simulink model "tqdtqr_rebuild_V3"  (R2021b)
settings: Solver=VariableStepAuto  StartTime=0.0  StopTime=10.0  RelTol=1e-3
undefined symbols (not defined in the file): ATQD_AfterTqMinGain_X_Deg, ATQD_APSCreepBaseTqD_X_kph, ATQD_APSCreepBaseTqD_Y_Deg, ATQD_APSCreepBaseTqR_X_kph, ATQD_APSCreepBaseTqR_Y_Deg, ATQD_APSCreepIterm_X_kph, ATQD_APSCreepIterm_Y_kph, ATQD_APSCreepPterm_X_kph, ATQD_APSCreepPterm_Y_kph, ATQD_APSDecReq_X_kph, ATQD_APSDecReq_Y_mps2, ATQD_APSDecReqCMD_X_kph, ATQD_APSDecReqTs_X_pct, ATQD_APSDecTimeGain_X_Deg, ATQD_APSDecTimeGain_Y_s, ATQD_APSReqLowSpd_X_Deg, ATQD_AutoHoldReleaseBPS_X_Deg, ATQD_AWDLoadTrqnsGain_X_kg, ATQD_AWDLoadTrqnsGain_Y_pct, ATQD_BOSEnBPSPosn_X_kph, ATQD_BOSMap_X_rpm, ATQD_BOSMap_Y_pct, ATQD_CreepBaseTqD_X_kph, ATQD_CreepBaseTqD_Y_Deg, ATQD_CreepBaseTqR_X_kph, ATQD_CreepBaseTqR_Y_Deg, ATQD_CreepBPSDisPosn_X_Deg, ATQD_CreepBPSDisPosnR_X_Deg, ATQD_CreepBPSEnPosn_X_Deg, ATQD_CreepBPSEnPosnR_X_Deg, ATQD_CreepDeltaTq_X_kph, ATQD_CreepIterm_X_kph, ATQD_CreepIterm_Y_kph, ATQD_CreepItermMaxLimit_X_pct, ATQD_CreepPreloadTime_X_kph, ATQD_CreepPreloadTq_X_kph, ATQD_CreepPreloadTq_Y_s, ATQD_CreepProtTq_X_Deg, ATQD_CreepPterm_X_kph, ATQD_CreepPterm_Y_kph, ATQD_CreepRrTqSpRat_X_rpm, ATQD_CreepRrTqSpRat_Y_Nm, ATQD_CreepTargetSpdD_X_pct, ATQD_CreepTargetSpdR_X_pct, ATQD_CreepUpLimitTq_X_rpm, ATQD_DecIneOPDHoldEnDelay_X_Deg, ATQD_DecIneOPDHoldEnDelay_Y_bar, ATQD_ECOTqMapD_X_rpm, ATQD_ECOTqMapD_Y_pct, ATQD_EMTqMapD_X_rpm, ATQD_EMTqMapD_Y_pct, ATQD_EOPDTqMapDCon_X_rpm, ATQD_EOPDTqMapDCon_Y_Deg, ATQD_EstInitVehWeight_X_c, ATQD_FAfterTqCMDGain_X_rpm, ATQD_FAfterTqCMDGain_Y_pct, ATQD_ForceLowSpd_X_Deg, ATQD_ForcePLimitSpd_X_Deg, ATQD_FrLossMAPLowV_X_rpm, ATQD_FrLossMAPLowV_Y_Nm ... (+949)
libraries: simulink x235, hcu_lib x208, tqr x63, tqd x6
(part 20 of 37)

== system tqdtqr_rebuild_V3/Input_Convert/Main function/Front//Rear ramp parameters determine/Rear First order filter input tau map and determination ==
  note: Drive mode case
  note: Determine Tq by different case
  VTQD_TqTargetShaftSpd_rpm : Inport
  VTQR_EVDriveMode_enum : Inport  Port=2
  VTQD_RollRegenEnable_flg : Inport  Port=3
  VTQD_TqSourceRr_enum : Inport  Port=4
  VTQR_REDUWhlTqReqSmooth_Nm : Inport  Port=5
  VDHP_ActAPSPosn_pct : Inport  Port=6
  VINP_VehSpeed_kph : Inport  Port=7
  VTQD_LimpHomeAct_flg : Inport  Port=8
  VTQD_EVDriveModeValid_flg : Inport  Port=9
  VTQD_RegenMode_enum : Inport  Port=10
  VVMC_ACCPedalOvrd_flg : Inport  Port=11
  VVMC_CCPedalOvrd_flg : Inport  Port=12
  VTQD_PreLoadHold_flg : Inport  Port=13
  VVMC_ActMaxSlideRate_pct : Inport  Port=14
  VTQD_CreepPrLoadEnable_flg : Inport  Port=15
  VTQD_RDCActive_enum : Inport  Port=16
  VTQR_NoABSREDUWhlTqReq_Nm : Inport  Port=17
  VTQR_RampREDUWhlTqReq_Nm : Inport  Port=18
  VTQR_RrFirstOrderInpTq_Nm : Inport  Port=19
  VTQD_PedAccTqEn_flg : Inport  Port=20
  VTQD_PreLoadPreEn_flg : Inport  Port=21
  VVMC_MSAWhlTqActive_flg : Inport  Port=22
  VINP_RrPTCSActive_flg : Inport  Port=23
  VINP_IVISnowModeCmd_flg : Inport  Port=24
  VTQD_IVIRockModeEn_flg : Inport  Port=25
  VINP_VehicleType_enum : Inport  Port=26
  VTQD_CoordWhlTqDemRr_Nm : Inport  Port=27
  VINP_RearAxlTrqReqDrv_Nm : Inport  Port=28
  VVMC_EstSlope_Deg : Inport  Port=29
  AND : Logic  AllPortsSameDT=off  OutDataTypeStr=boolean
  AND1 : Logic  Inputs=3  AllPortsSameDT=off  OutDataTypeStr=boolean
  AND2 : Logic  Inputs=3  AllPortsSameDT=off  OutDataTypeStr=boolean
  AND3 : Logic  AllPortsSameDT=off  OutDataTypeStr=boolean
  AND4 : Logic  AllPortsSameDT=off  OutDataTypeStr=boolean
  Abs : Abs
  Abs4 : Abs
  Add : Sum  Inputs=+-
  Add1 : Sum  Inputs=+-
  Constant1 : Constant  Value=ENUM_TQSOURCE_APS
  Constant10 : Constant  Value=KTQR_PreLoadTs_c
  Constant12 : Constant  Value=KTQR_ARegenLatchEnTq_Nm
  Constant13 : Constant  Value=KTQR_PreLoadPreEnTs_c
  Constant18 : Constant  Value=ENUM_DRIVEMODE_ECO
  Constant19 : Constant  Value=ENUM_DRIVEMODE_NRM
  Constant2 : Constant  Value=KTQR_DriveModeChangeTq_Nm
  Constant20 : Constant  Value=ENUM_DRIVEMODE_SPORT
  Constant3 : Constant  Value=ENUM_TQSOURCE_CC
  Constant32 : Constant  Value=KTQR_TIPOutTsAPS_pct
  Constant33 : Constant  Value=KTQR_TIPOutTsSpd_kph
  Constant34 : Constant  Value=ENUM_TQSOURCE_ADAS
  Constant5 : Constant  Value=ENUM_RDCACTSTA_NOREQUEST
  Constant7 : Constant  Value=ENUM_TQSOURCE_MSA
  Constant8 : Constant  Value=KTQR_DriveModeCMDTqDev_Nm
  Constant9 : Constant  Value=ENUM_VEHICLETYPE_D31L24
  Delay : Delay  DelayLength=1
  Delay1 : Delay  DelayLength=1
  Delay2 : Delay  DelayLength=1
  Detect Change : simulink/Logic and Bit Operations/Detect Change  vinit=0  OutDataTypeStr=boolean
  Equal16 : RelationalOperator  Operator===  OutDataTypeStr=boolean  RndMeth=Simplest
  Equal17 : RelationalOperator  Operator===  OutDataTypeStr=boolean  RndMeth=Simplest
  Equal19 : RelationalOperator  Operator===  OutDataTypeStr=boolean  RndMeth=Simplest
  Equal2 : RelationalOperator  Operator=~=  OutDataTypeStr=boolean  RndMeth=Simplest
  Equal6 : RelationalOperator  Operator=~=  OutDataTypeStr=boolean  RndMeth=Simplest
  GreaterThan2 : RelationalOperator  OutDataTypeStr=boolean  RndMeth=Simplest
  If : If  NumInputs=7  IfExpression=u1~= 0  ElseIfExpressions=u2 ~= 0, u3 ~= 0,u4 ~= 0,u5 ~= 0,u6 ~= 0
  If1 : If  NumInputs=6  IfExpression=u1~= 0  ElseIfExpressions=u2 ~= 0, u3 ~= 0,u4~=0,u5~=0,u6~=0
  Less Than2 : RelationalOperator  Operator=<=  OutDataTypeStr=boolean  RndMeth=Simplest
  Logical Operator : Logic  AllPortsSameDT=off  OutDataTypeStr=boolean
  Logical Operator1 : Logic  Inputs=3  AllPortsSameDT=off  OutDataTypeStr=boolean
  Logical Operator14 : Logic  Operator=OR  Inputs=5  AllPortsSameDT=off  OutDataTypeStr=boolean
  Logical Operator2 : Logic  AllPortsSameDT=off  OutDataTypeStr=boolean
  Logical Operator3 : Logic  Operator=NOT  AllPortsSameDT=off  OutDataTypeStr=boolean
  Logical Operator8 : Logic  Operator=OR  AllPortsSameDT=off  OutDataTypeStr=boolean
  Logical Operator9 : Logic  Operator=NOT  AllPortsSameDT=off  OutDataTypeStr=boolean
  Merge : Merge  Inputs=7
  Merge3 : Merge  Inputs=7
  NOT : Logic  Operator=NOT  AllPortsSameDT=off  OutDataTypeStr=boolean
  NOT1 : Logic  Operator=NOT  AllPortsSameDT=off  OutDataTypeStr=boolean
  OR2 : Logic  Operator=OR  AllPortsSameDT=off  OutDataTypeStr=boolean
  Relational Operator : RelationalOperator  Operator=>  OutDataTypeStr=boolean  RndMeth=Simplest
  Relational Operator1 : RelationalOperator  Operator=~=  OutDataTypeStr=boolean  RndMeth=Simplest
  Relational Operator2 : RelationalOperator  Operator=<=  OutDataTypeStr=boolean  RndMeth=Simplest
  Relational Operator3 : RelationalOperator  Operator===  OutDataTypeStr=boolean  RndMeth=Simplest
  Relational Operator4 : RelationalOperator  Operator===  OutDataTypeStr=boolean  RndMeth=Simplest
  Relational Operator5 : RelationalOperator  Operator=<  OutDataTypeStr=boolean  RndMeth=Simplest
  Relational Operator6 : RelationalOperator  OutDataTypeStr=boolean  RndMeth=Simplest
  Relational Operator7 : RelationalOperator  Operator===  OutDataTypeStr=boolean  RndMeth=Simplest
  SR_Latch1 : hcu_lib/Basic_Blocks/SR_Latch
  Switch4 : Switch  Criteria=u2 > Threshold
  VTQR_CreepREDUTs_c : Subsystem  TreatAsAtomicUnit=on
  VTQR_ECOREDUTs_c : tqr/TQR/Determine Torque Request/TorqueArbitrament/TorqueSmooth/Rear First order filter input tau map and determination/VTQR_ECOREDUTs_c  SystemSampleTime=-1  VariantActivationTime=update diagram  Latency=0  AutoFrameSizeCalculation=off
  VTQR_ESCAPEREDUTs_c : tqr/TQR/Determine Torque Request/TorqueArbitrament/TorqueSmooth/Rear First order filter input tau map and determination/VTQR_ESCAPEREDUTs_c  SystemSampleTime=-1  VariantActivationTime=update diagram  Latency=0  AutoFrameSizeCalculation=off
  VTQR_LHMREDUTs_c : tqr/TQR/Determine Torque Request/TorqueArbitrament/TorqueSmooth/Rear First order filter input tau map and determination/VTQR_LHMREDUTs_c  SystemSampleTime=-1  VariantActivationTime=update diagram  Latency=0  AutoFrameSizeCalculation=off
  VTQR_NORMALREDUTs_c : tqr/TQR/Determine Torque Request/TorqueArbitrament/TorqueSmooth/Rear First order filter input tau map and determination/VTQR_NORMALREDUTs_c  SystemSampleTime=-1  VariantActivationTime=update diagram  Latency=0  AutoFrameSizeCalculation=off
  VTQR_PreLoadPreEnTs_c : Subsystem  TreatAsAtomicUnit=on
  VTQR_PreLoadTs_c : Subsystem  TreatAsAtomicUnit=on
  VTQR_RDCActiveREDUTs_c : Subsystem  TreatAsAtomicUnit=on
  VTQR_REDUTIPOutTs_c : Subsystem  TreatAsAtomicUnit=on
  VTQR_REDUTs_c : Subsystem  TreatAsAtomicUnit=on
  VTQR_SNOWREDUTs_c : tqr/TQR/Determine Torque Request/TorqueArbitrament/TorqueSmooth/Rear First order filter input tau map and determination/VTQR_SNOWREDUTs_c  SystemSampleTime=-1  VariantActivationTime=update diagram  Latency=0  AutoFrameSizeCalculation=off
  VTQR_SPORTREDUTs_c : tqr/TQR/Determine Torque Request/TorqueArbitrament/TorqueSmooth/Rear First order filter input tau map and determination/VTQR_SPORTREDUTs_c  SystemSampleTime=-1  VariantActivationTime=update diagram  Latency=0  AutoFrameSizeCalculation=off
  VTQR_TCSREDUTs_c : tqr/TQR/Determine Torque Request/TorqueArbitrament/TorqueSmooth/Rear First order filter input tau map and determination/VTQR_TCSREDUTs_c  SystemSampleTime=-1  VariantActivationTime=update diagram  Latency=0  AutoFrameSizeCalculation=off
  VTQR_VMCREDUTs_c : Subsystem  TreatAsAtomicUnit=on
  VTQR_RrFirstOrderInpTs_c : Outport
  wires:
  VINP_RearAxlTrqReqDrv_Nm/1 -> [VINP_RearAxlTrqReqDrv_Nm]
  VTQD_CoordWhlTqDemRr_Nm/1 -> [VTQD_CoordWhlTqDemRr_Nm]
  VINP_VehicleType_enum/1 -> [VINP_VehicleType_enum]
  VINP_IVISnowModeCmd_flg/1 -> [VINP_IVISnowModeCmd_flg]
  VTQD_IVIRockModeEn_flg/1 -> [VTQD_IVIRockModeEn_flg]
  VINP_RrPTCSActive_flg/1 -> [VINP_RrPTCSActive_flg]
  [VTQD_PedAccTqEn_flg] -> Logical Operator14/5
  VVMC_MSAWhlTqActive_flg/1 -> [VVMC_MSAWhlTqActive_flg]
  AND3/1 -> Logical Operator14/4
  [VTQD_TqSourceRr_enum] -> Relational Operator7/1
  Relational Operator7/1 -> AND3/1
  Constant7/1 -> Relational Operator7/2
  [VVMC_MSAWhlTqActive_flg] -> AND3/2
  VTQD_PreLoadPreEn_flg/1 -> [VTQD_PreLoadPreEn_flg]
  VVMC_ActMaxSlideRate_pct/1 -> [VVMC_ActMaxSlideRate_pct]
  VTQD_PedAccTqEn_flg/1 -> [VTQD_PedAccTqEn_flg]
  VTQR_RrFirstOrderInpTq_Nm/1 -> [VTQR_RrFirstOrderInpTq_Nm]
  VTQR_RampREDUWhlTqReq_Nm/1 -> [VTQR_RampREDUWhlTqReq_Nm]
  VTQR_NoABSREDUWhlTqReq_Nm/1 -> [VTQR_NoABSREDUWhlTqReq_Nm]
  VTQD_RDCActive_enum/1 -> [VTQD_RDCActive_enum]
  Relational Operator2/1 -> AND/1
  AND/1 -> [VTQR_RrRDCActiveTs_flg]  "VTQR_RrRDCActiveTs_flg"
  Constant5/1 -> Equal2/2
  Equal2/1 -> AND/2
  [VTQD_RDCActive_enum] -> Equal2/1
  [VTQR_RampREDUWhlTqReq_Nm] -> Relational Operator2/1
  Constant12/1 -> Relational Operator2/2
  [VTQD_CreepPrLoadEnable_flg] -> Logical Operator14/3
  VTQD_CreepPrLoadEnable_flg/1 -> [VTQD_CreepPrLoadEnable_flg]
  VTQD_PreLoadHold_flg/1 -> [VTQD_PreLoadHold_flg]
  Constant32/1 -> Less Than2/2
  [VDHP_ActAPSPosn_pct] -> Less Than2/1
  [VTQD_TqSourceRr_enum] -> Relational Operator3/1
  [VVMC_ACCPedalOvrd_flg] -> NOT/1
  [VVMC_CCPedalOvrd_flg] -> NOT1/1
  Relational Operator1/1 -> AND2/3
  Logical Operator14/1 -> AND1/1
  Constant1/1 -> Relational Operator1/2
  GreaterThan2/1 -> AND2/2
  Constant33/1 -> GreaterThan2/2
  NOT/1 -> AND1/2
  NOT1/1 -> AND1/3
  [VTQD_TqSourceRr_enum] -> Relational Operator1/1
  Less Than2/1 -> AND2/1
  [VTQD_TqSourceRr_enum] -> Relational Operator4/1
  Constant34/1 -> Relational Operator4/2
  Relational Operator4/1 -> Logical Operator14/2
  [VINP_VehSpeed_kph] -> GreaterThan2/1
  Relational Operator3/1 -> Logical Operator14/1
  Constant3/1 -> Relational Operator3/2
  VVMC_CCPedalOvrd_flg/1 -> [VVMC_CCPedalOvrd_flg]
  VVMC_ACCPedalOvrd_flg/1 -> [VVMC_ACCPedalOvrd_flg]
  VTQD_RegenMode_enum/1 -> [VTQD_RegenMode_enum]
  VTQD_EVDriveModeValid_flg/1 -> [VTQD_EVDriveModeValid_flg]
  VTQD_RollRegenEnable_flg/1 -> [VTQD_RollRegenEnable_flg]
  VINP_VehSpeed_kph/1 -> [VINP_VehSpeed_kph]
  VDHP_ActAPSPosn_pct/1 -> [VDHP_ActAPSPosn_pct]
  VTQD_LimpHomeAct_flg/1 -> [VTQD_LimpHomeAct_flg]
  VTQR_REDUWhlTqReqSmooth_Nm/1 -> [VTQR_REDUWhlTqReqSmooth_Nm]
  VTQD_TqSourceRr_enum/1 -> [VTQD_TqSourceRr_enum]
  VTQD_TqTargetShaftSpd_rpm/1 -> [VTQD_TqTargetShaftSpd_rpm]
  VTQR_EVDriveMode_enum/1 -> [VTQR_EVDriveMode_enum]
  AND1/1 -> [VTQD_ADASCreepCondition_flg]
  AND2/1 -> [VTQD_APSCondition_flg]
  [VTQR_RrRDCActiveTs_flg] -> If1/1
  If1/1 -> VTQR_RDCActiveREDUTs_c/Action
  [VTQD_RegenMode_enum] -> VTQR_RDCActiveREDUTs_c/1(VTQD_RegenMode_enum)
  [VVMC_ActMaxSlideRate_pct] -> VTQR_RDCActiveREDUTs_c/2(VVMC_ActMaxSlideRate_pct)
  If1/2 -> VTQR_CreepREDUTs_c/Action
  Logical Operator/1 -> If1/2
  [VTQD_ADASCreepCondition_flg] -> Logical Operator/1
  [VTQD_CreepPrLoadEnable_flg] -> Logical Operator/2
  [VTQR_REDUWhlTqReqSmooth_Nm] -> VTQR_CreepREDUTs_c/1(VTQR_REDUWhlTqReqSmooth_Nm)
  [VTQD_TqTargetShaftSpd_rpm] -> VTQR_CreepREDUTs_c/2(VTQD_TqTargetShaftSpd_rpm)
  [VTQD_ADASCreepCondition_flg] -> Logical Operator2/1
  Logical Operator2/1 -> If1/3
  [VTQD_CreepPrLoadEnable_flg] -> Logical Operator3/1
  Logical Operator3/1 -> Logical Operator2/2
  If1/3 -> VTQR_VMCREDUTs_c/Action
  [VTQR_REDUWhlTqReqSmooth_Nm] -> VTQR_VMCREDUTs_c/1(VTQR_REDUWhlTqReqSmooth_Nm)
  [VTQD_TqTargetShaftSpd_rpm] -> VTQR_VMCREDUTs_c/2(VTQD_TqTargetShaftSpd_rpm)
  [VTQD_APSCondition_flg] -> If1/4
  If1/4 -> VTQR_REDUTIPOutTs_c/Action
  [VTQD_PreLoadHold_flg] -> If1/5
  Constant13/1 -> VTQR_PreLoadPreEnTs_c/1(KTQR_PreLoadPreEnTs_c)
  [VTQD_TqTargetShaftSpd_rpm] -> VTQR_REDUTIPOutTs_c/1(VTQD_TqTargetShaftSpd_rpm)
  [VTQD_PreLoadPreEn_flg] -> If1/6
  If1/6 -> VTQR_PreLoadPreEnTs_c/Action
  Constant10/1 -> VTQR_PreLoadTs_c/1(KTQR_PreLoadTs_c)
  If1/5 -> VTQR_PreLoadTs_c/Action
  VTQR_RDCActiveREDUTs_c/1(VTQR_RDCActiveREDUTs_c) -> [VTQR_RDCActiveREDUTs_c]  "VTQR_RDCActiveREDUTs_c"
  VTQR_CreepREDUTs_c/1(VTQR_CreepREDUTs_c) -> [VTQR_CreepREDUTs_c]  "VTQR_CreepREDUTs_c"
  VTQR_VMCREDUTs_c/1(VTQR_VMCREDUTs_c) -> [VTQR_VMCREDUTs_c]  "VTQR_VMCREDUTs_c"
  VTQR_REDUTIPOutTs_c/1(VTQR_REDUTIPOutTs_c) -> [VTQR_REDUTIPOutTs_c]  "VTQR_REDUTIPOutTs_c"
  VTQR_PreLoadTs_c/1(VTQR_PreLoadTs_c) -> [VTQR_PreLoadTs_c]  "VTQR_PreLoadTs_c"
  VTQR_PreLoadPreEnTs_c/1(VTQR_PreLoadPreEnTs_c) -> [VTQR_PreLoadPreEnTs_c]  "VTQR_PreLoadPreEnTs_c"
  [VTQR_REDUTIPOutTs_c] -> Merge/4
  [VTQR_PreLoadTs_c] -> Merge/5
  [VTQR_PreLoadPreEnTs_c] -> Merge/6
  [VTQR_VMCREDUTs_c] -> Merge/3
  [VTQR_CreepREDUTs_c] -> Merge/2
  [VTQR_RDCActiveREDUTs_c] -> Merge/1
  Merge/1 -> VTQR_RrFirstOrderInpTs_c/1  "VTQR_RrFirstOrderInpTs_c"
  VTQR_SNOWREDUTs_c/1 -> [VTQR_SNOWREDUTs_c]  "VTQR_SNOWREDUTs_c"
  Relational Operator/1 -> Logical Operator1/3
  VTQR_NORMALREDUTs_c/1 -> [VTQR_NORMALREDUTs_c]  "VTQR_NORMALREDUTs_c"
  Equal6/1 -> Logical Operator1/2
  [VINP_RearAxlTrqReqDrv_Nm] -> Relational Operator/2
  VTQR_ESCAPEREDUTs_c/1 -> [VTQR_ESCAPEREDUTs_c]  "VTQR_ESCAPEREDUTs_c"
  Logical Operator1/1 -> If/2
  If/5 -> VTQR_NORMALREDUTs_c/Action
  Equal16/1 -> If/6
  [VTQR_REDUWhlTqReqSmooth_Nm] -> VTQR_NORMALREDUTs_c/1
  VTQR_TCSREDUTs_c/1 -> [VTQR_TCSREDUTs_c]  "VTQR_TCSREDUTs_c"
  [VINP_IVISnowModeCmd_flg] -> If/4
  Equal17/1 -> If/5
  Constant18/1 -> Equal16/2
  [VINP_VehicleType_enum] -> Equal6/1
  [VTQD_IVIRockModeEn_flg] -> If/3
  VTQR_LHMREDUTs_c/1 -> [VTQR_LHMREDUTs_c]  "VTQR_LHMREDUTs_c"
  Logical Operator8/1 -> If/1
  VTQR_SPORTREDUTs_c/1 -> [VTQR_SPORTREDUTs_c]  "VTQR_SPORTREDUTs_c"
  If/7 -> VTQR_SPORTREDUTs_c/Action
  [VTQR_REDUWhlTqReqSmooth_Nm] -> VTQR_SNOWREDUTs_c/1
  [VTQR_EVDriveMode_enum] -> Equal17/1
  If/4 -> VTQR_SNOWREDUTs_c/Action
  VTQR_ECOREDUTs_c/1 -> [VTQR_ECOREDUTs_c]  "VTQR_ECOREDUTs_c"
  [VTQD_CoordWhlTqDemRr_Nm] -> Relational Operator/1
  [VTQD_TqTargetShaftSpd_rpm] -> VTQR_SPORTREDUTs_c/2
  [VTQR_REDUWhlTqReqSmooth_Nm] -> VTQR_TCSREDUTs_c/1
  [VTQD_RollRegenEnable_flg] -> VTQR_ECOREDUTs_c/4
  [VTQD_TqTargetShaftSpd_rpm] -> VTQR_TCSREDUTs_c/2
  [VTQD_RegenMode_enum] -> VTQR_NORMALREDUTs_c/3
  [VTQD_TqTargetShaftSpd_rpm] -> VTQR_NORMALREDUTs_c/2
  If/3 -> VTQR_ESCAPEREDUTs_c/Action
  Constant20/1 -> Equal19/2
  [VTQD_TqTargetShaftSpd_rpm] -> VTQR_ESCAPEREDUTs_c/2
  [VTQR_REDUWhlTqReqSmooth_Nm] -> VTQR_ESCAPEREDUTs_c/1
  [VTQR_EVDriveMode_enum] -> Equal16/1
  If/6 -> VTQR_ECOREDUTs_c/Action
  [VINP_RrPTCSActive_flg] -> Logical Operator1/1
  [VTQD_RegenMode_enum] -> VTQR_SPORTREDUTs_c/3
  [VTQR_REDUWhlTqReqSmooth_Nm] -> VTQR_SPORTREDUTs_c/1
  [VTQD_RegenMode_enum] -> VTQR_ECOREDUTs_c/3
  Equal19/1 -> If/7
  Logical Operator9/1 -> Logical Operator8/2
  [VTQD_TqTargetShaftSpd_rpm] -> VTQR_SNOWREDUTs_c/2
  [VTQR_REDUWhlTqReqSmooth_Nm] -> VTQR_ECOREDUTs_c/1
  [VTQR_REDUWhlTqReqSmooth_Nm] -> VTQR_LHMREDUTs_c/1
  If/1 -> VTQR_LHMREDUTs_c/Action
  [VTQR_EVDriveMode_enum] -> Equal19/1
  [VTQD_TqTargetShaftSpd_rpm] -> VTQR_LHMREDUTs_c/2
  Constant9/1 -> Equal6/2
  [VTQD_EVDriveModeValid_flg] -> Logical Operator9/1
  Constant19/1 -> Equal17/2
  If/2 -> VTQR_TCSREDUTs_c/Action
  [VTQD_TqTargetShaftSpd_rpm] -> VTQR_ECOREDUTs_c/2
  [VTQD_LimpHomeAct_flg] -> Logical Operator8/1
  [VTQR_NORMALREDUTs_c] -> Merge3/5
  Merge3/1 -> Switch4/3
  [VTQR_ECOREDUTs_c] -> Merge3/6
  [VTQR_LHMREDUTs_c] -> Merge3/1
  [VTQR_SNOWREDUTs_c] -> Merge3/4
  [VTQR_RrDrModChangeReset_flg] -> SR_Latch1/2
  SR_Latch1/1 -> Switch4/2, [VTQR_RrDrModTsLatch_flg]  "VTQR_RrDrModLatch_flg"
  [VTQR_EVDriveMode_enum] -> Detect Change/1
  Detect Change/1 -> SR_Latch1/1
  [VTQR_SPORTREDUTs_c] -> Merge3/7
  Delay/1 -> Switch4/1
  [VTQR_TCSREDUTs_c] -> Merge3/2
  Switch4/1 -> [VTQR_REDUTs_c], Delay/1  "VTQR_REDUTs_c"
  [VTQR_ESCAPEREDUTs_c] -> Merge3/3
  Relational Operator5/1 -> OR2/1
  Add/1 -> Abs/1
  Delay2/1 -> AND4/2
  Constant8/1 -> Relational Operator6/2
  Add1/1 -> Abs4/1
  [VTQR_RrFirstOrderInpTq_Nm] -> Add1/2
  [VTQR_RrFirstOrderInpTq_Nm] -> Add/2
  [VTQR_NoABSREDUWhlTqReq_Nm] -> Add/1
  [VTQR_RrDrModTsLatch_flg] -> Delay2/1
  Relational Operator6/1 -> AND4/1
  OR2/1 -> [VTQR_RrDrModChangeReset_flg]
  Constant2/1 -> Relational Operator5/2
  Abs/1 -> Relational Operator5/1
  [VTQR_RrFirstOrderInpTq_Nm] -> Delay1/1
  AND4/1 -> OR2/2
  Abs4/1 -> Relational Operator6/1
  Delay1/1 -> Add1/1
  If1/7 -> VTQR_REDUTs_c/Action
  [VTQR_REDUTs_c] -> VTQR_REDUTs_c/1(VTQR_REDUTs_c)
  VTQR_REDUTs_c/1(VTQR_OutREDUTs_c) -> [VTQR_OutREDUTs_c]  "VTQR_OutREDUTs_c"
  [VTQR_OutREDUTs_c] -> Merge/7
  VVMC_EstSlope_Deg/1 -> [VVMC_EstSlope_Deg]
  [VVMC_EstSlope_Deg] -> VTQR_CreepREDUTs_c/3(VVMC_EstSlope_Deg)

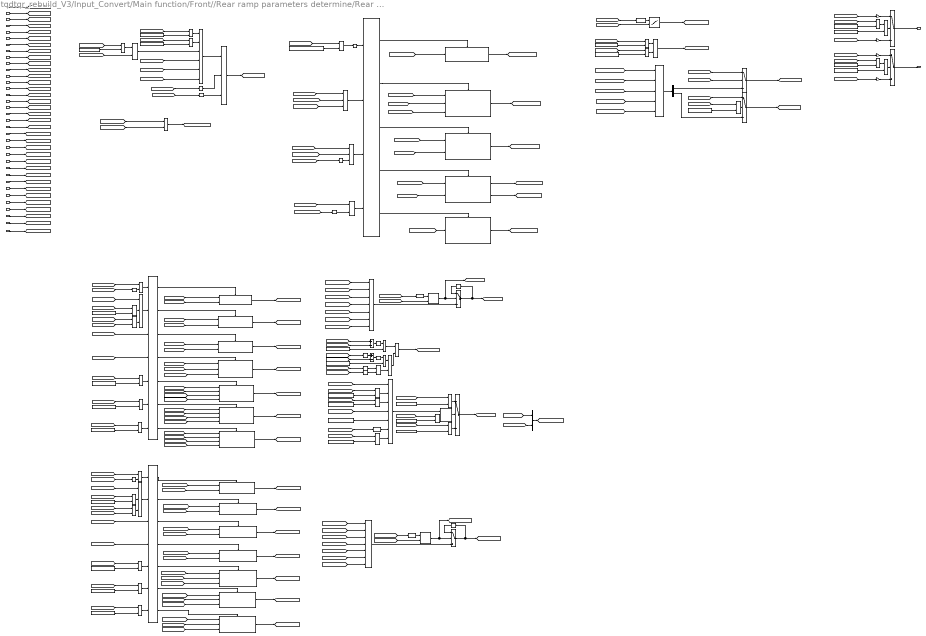
== system tqdtqr_rebuild_V3/Input_Convert/Main function/Front//Rear ramp parameters determine/Rear wheel rate limit determination1 ==
  note: Drive mode case
  note: Determin torque by different cases
  note: Check direction
  note: Merge result and decide final Tq
  VTQR_RrTqZeroTrans_enum : Inport
  VTQD_TqSourceRr_enum : Inport  Port=2
  VTQD_TqTargetShaftSpd_rpm : Inport  Port=3
  VTQD_LimpHomeAct_flg : Inport  Port=4
  VTQR_EVDriveMode_enum : Inport  Port=5
  VDHP_ActAPSPosn_pct : Inport  Port=6
  VTQR_REDUWhlTqReqSmoothDelay_Nm : Inport  Port=7
  VTQD_EVDriveModeValid_flg : Inport  Port=8
  VTQD_RegenMode_enum : Inport  Port=9
  VVMC_ACCPedalOvrd_flg : Inport  Port=10
  VVMC_CCPedalOvrd_flg : Inport  Port=11
  VTQD_CreepPrLoadEnable_flg : Inport  Port=12
  VTQD_RegenTqLimitEn_flg : Inport  Port=13
  VTQD_RDCActive_enum : Inport  Port=14
  VTQD_PreLoadPreEn_flg : Inport  Port=15
  VTQR_NoABSREDUWhlTqReq_Nm : Inport  Port=16
  VTQR_RampREDUWhlTqReq_Nm : Inport  Port=17
  VTQR_RrFirstOrderInpTq_Nm : Inport  Port=18
  VVMC_ActMaxSlideRate_pct : Inport  Port=19
  VTQD_PedAccTqEn_flg : Inport  Port=20
  VVMC_MSAWhlTqActive_flg : Inport  Port=21
  VINP_RrPTCSActive_flg : Inport  Port=22
  VTQD_GearActualPosn_enum : Inport  Port=23
  VINP_IVISnowModeCmd_flg : Inport  Port=24
  VTQD_IVIRockModeEn_flg : Inport  Port=25
  VTQD_RrShaftSpd_rpm : Inport  Port=26
  VVMC_EstSlope_Deg : Inport  Port=27
  VTQD_VehActSpd_kph : Inport  Port=28
  VINP_ACCVehHoldReq_flg : Inport  Port=29
  VPMM_DriveTrainSelect_enum : Inport  Port=30
  VVMC_ADASActive_flg : Inport  Port=31
  VINP_VehicleType_enum : Inport  Port=32
  VTQD_CoordWhlTqDemRr_Nm : Inport  Port=33
  VINP_RearAxlTrqReqDrv_Nm : Inport  Port=34
  VTQD_RrZeroPointIncDec_Nm : Inport  Port=35
  " Relational Operator1" : RelationalOperator  Operator=>  OutDataTypeStr=boolean  RndMeth=Simplest
  " Relational Operator8" : RelationalOperator  Operator=>  OutDataTypeStr=boolean  RndMeth=Simplest
  AND{,2,4..6,9} (6 alike) : Logic  AllPortsSameDT=off  OutDataTypeStr=boolean
  AND7 : Logic  Inputs=7  AllPortsSameDT=off  OutDataTypeStr=boolean
  AND8 : Logic  Inputs=3  AllPortsSameDT=off  OutDataTypeStr=boolean
  Abs : Abs
  Abs4 : Abs
  Add : Sum  Inputs=+-
  Add1 : Sum  Inputs=+-
  Constant : Constant  Value=KTQR_ACCHoldPdovrdGrade_Deg
  Constant11 : Constant  Value=KTQR_ACCHoldPdovrdVeh_kph
  Constant12 : Constant  Value=KTQR_ARegenLatchEnTq_Nm
  Constant13 : Constant  Value=KTQR_ACCHoldPdovrdSW_flg
  Constant14 : Constant  Value=ENUM_DRIVETRAIN_RWD
  Constant15 : Constant  Value=KTQR_ACCHoldPdovrdInc_Nm
  Constant16 : Constant  Value=KTQR_ACCHoldPdovrdInc_Nm
  Constant17 : Constant  Value=ZERO_FLOAT
  Constant18 : Constant  Value=ENUM_GEARACTUALPOSN_R
  Constant19 : Constant  Value=KTQR_NewRampArchSW_flg
  Constant2 : Constant  Value=KTQR_DriveModeChangeTq_Nm
  Constant20 : Constant  Value=ENUM_GEARACTUALPOSN_R
  Constant21 : Constant  Value=KTQR_NewRampArchSW_flg
  Constant22 : Constant  Value=ENUM_DRIVEMODE_ECO
  Constant23 : Constant  Value=ENUM_DRIVEMODE_NRM
  Constant24 : Constant  Value=ENUM_DRIVEMODE_SPORT
  Constant25 : Constant  Value=ENUM_VEHICLETYPE_D31L24
  Constant26 : Constant  Value=ENUM_DRIVEMODE_ECO
  Constant27 : Constant  Value=ENUM_DRIVEMODE_NRM
  Constant28 : Constant  Value=ENUM_DRIVEMODE_SPORT
  Constant29 : Constant  Value=ENUM_VEHICLETYPE_D31L24
  Constant30 : Constant  Value=ENUM_TQSOURCE_ADAS
  Constant4 : Constant  Value=ENUM_TQZEROTRANS_NOZEROTRANS
  Constant5 : Constant  Value=ENUM_RDCACTSTA_NOREQUEST
  Constant6 : Constant  Value=KTQR_RegenTqLimitDecSW_flg
  Constant7 : Constant  Value=ENUM_TQSOURCE_MSA
  Constant8 : Constant  Value=KTQR_DriveModeCMDTqDev_Nm
  Constant9 : Constant  Value=ENUM_TQSOURCE_CC
  Data Type Conversion : DataTypeConversion  OutDataTypeStr=single
  Delay{,1..4} (5 alike) : Delay  DelayLength=1
  Demux : Demux  Outputs=2
  Detect Change : simulink/Logic and Bit Operations/Detect Change  vinit=0  OutDataTypeStr=boolean
  Detect Change1 : simulink/Logic and Bit Operations/Detect Change  vinit=0  OutDataTypeStr=boolean
  Detect Increase : simulink/Logic and Bit Operations/Detect Increase  vinit=0.0  OutDataTypeStr=boolean
  Drive mode : Subsystem  TreatAsAtomicUnit=on
  Equal{,1,5,20..21,23..25,27} (9 alike) : RelationalOperator  Operator===  OutDataTypeStr=boolean  RndMeth=Simplest
  Equal2 : RelationalOperator  Operator=~=  OutDataTypeStr=boolean  RndMeth=Simplest
  Equal3 : RelationalOperator  OutDataTypeStr=boolean  RndMeth=Simplest
  Equal4 : RelationalOperator  Operator=<=  OutDataTypeStr=boolean  RndMeth=Simplest
  Equal6 : RelationalOperator  OutDataTypeStr=boolean  RndMeth=Simplest
  Equal7 : RelationalOperator  Operator=~=  OutDataTypeStr=boolean  RndMeth=Simplest
  Equal8 : RelationalOperator  Operator=~=  OutDataTypeStr=boolean  RndMeth=Simplest
  Gain2 : Gain
  Gain3 : Gain  Gain=-1
  Gain4 : Gain
  Gain5 : Gain  Gain=-1
  If3 : If  NumInputs=4  IfExpression=u1~= 0  ElseIfExpressions=u2 ~= 0, u3 ~= 0, u4~=0
  If4 : If  NumInputs=7  IfExpression=u1~= 0  ElseIfExpressions=u2 ~= 0, u3 ~= 0 ,u4 ~= 0, u5~=0, u6~=0, u7~=0  ShowElse=off
  If5 : If  NumInputs=7  IfExpression=u1~= 0  ElseIfExpressions=u2 ~= 0, u3 ~= 0,u4 ~= 0,u5 ~= 0,u6 ~= 0,u7 ~= 0  ShowElse=off
  Logical Operator{,1..2,5} (4 alike) : Logic  Inputs=3  AllPortsSameDT=off  OutDataTypeStr=boolean
  Logical Operator10 : Logic  Operator=OR  AllPortsSameDT=off  OutDataTypeStr=boolean
  Logical Operator{3,6,9,11,13} (5 alike) : Logic  Operator=NOT  AllPortsSameDT=off  OutDataTypeStr=boolean
  Logical Operator12 : Logic  Operator=OR  AllPortsSameDT=off  OutDataTypeStr=boolean
  Logical Operator4 : Logic  Operator=OR  Inputs=6  AllPortsSameDT=off  OutDataTypeStr=boolean
  Logical Operator8 : Logic  AllPortsSameDT=off  OutDataTypeStr=boolean
  MTQR_AltRDCActiveREDUInc_Z_Nm : Lookup_n-D  BreakpointsForDimension1=ATQR_AltRDCActiveREDUInc_Y_enum  BreakpointsForDimension2=ATQR_AltRDCActiveREDUInc_X_pct  Table=MTQR_AltRDCActiveREDUInc_Z_Nm  TableDataTypeStr=Inherit: Inherit from 'Table data'  ExtrapMethod=Clip  InternalRulePriority=Speed  RndMeth=Simplest  InputSameDT=on
      settings: InputPortMap=u0,u1
  Max : MinMax  Function=max  Inputs=2
  Max1 : MinMax  Function=max  Inputs=2
  Merge : Merge  Inputs=5
  Merge4 : Merge  Inputs=7
  Merge5 : Merge  Inputs=7
  Mux : Mux  Inputs=2
  NOT2 : Logic  Operator=NOT  AllPortsSameDT=off  OutDataTypeStr=boolean
  NOT3 : Logic  Operator=NOT  AllPortsSameDT=off  OutDataTypeStr=boolean
  OR1 : Logic  Operator=OR  AllPortsSameDT=off  OutDataTypeStr=boolean
  OR2 : Logic  Operator=OR  AllPortsSameDT=off  OutDataTypeStr=boolean
  OR3 : Logic  Operator=OR  AllPortsSameDT=off  OutDataTypeStr=boolean
  Relational Operator{1,8..10} (4 alike) : RelationalOperator  Operator===  OutDataTypeStr=boolean  RndMeth=Simplest
  Relational Operator2 : RelationalOperator  Operator=<=  OutDataTypeStr=boolean  RndMeth=Simplest
  Relational Operator5 : RelationalOperator  Operator=<  OutDataTypeStr=boolean  RndMeth=Simplest
  Relational Operator6 : RelationalOperator  OutDataTypeStr=boolean  RndMeth=Simplest
  SR_Latch1 : hcu_lib/Basic_Blocks/SR_Latch
  SR_Latch2 : hcu_lib/Basic_Blocks/SR_Latch
  SR_Latch3 : hcu_lib/Basic_Blocks/SR_Latch
  Switch{,7..10} (5 alike) : Switch  Criteria=u2 ~= 0
      Switch settings: AttributesFormatString=%<Criteria>
      Switch7 settings: AttributesFormatString=%<Criteria>
      Switch8 settings: AttributesFormatString=%<Criteria>
      Switch9 settings: AttributesFormatString=%<Criteria>
  Switch4 : Switch  Criteria=u2 > Threshold
  Switch5 : Switch  Criteria=u2 > Threshold
  VTQD_OutRrZeroPointIncDec_Nm : Subsystem  TreatAsAtomicUnit=on
  VTQR_CreepREDUTqIncDecSR_Nm : Subsystem  TreatAsAtomicUnit=on
  VTQR_ECOREDURateLimitDec_Nm : tqr/TQR/Determine Torque Request/TorqueArbitrament/TorqueSmooth/Rear wheel rate limit determination1/VTQR_ECOREDURateLimitDec_Nm  SystemSampleTime=-1  VariantActivationTime=update diagram  Latency=0  AutoFrameSizeCalculation=off
  VTQR_ECOREDURateLimitInc_Nm : tqr/TQR/Determine Torque Request/TorqueArbitrament/TorqueSmooth/Rear wheel rate limit determination1/VTQR_ECOREDURateLimitInc_Nm  SystemSampleTime=-1  VariantActivationTime=update diagram  Latency=0  AutoFrameSizeCalculation=off
  VTQR_ESCAPEREDURateLimitDec_Nm : tqr/TQR/Determine Torque Request/TorqueArbitrament/TorqueSmooth/Rear wheel rate limit determination1/VTQR_ESCAPEREDURateLimitDec_Nm  SystemSampleTime=-1  VariantActivationTime=update diagram  Latency=0  AutoFrameSizeCalculation=off
  VTQR_ESCAPEREDURateLimitInc_Nm : tqr/TQR/Determine Torque Request/TorqueArbitrament/TorqueSmooth/Rear wheel rate limit determination1/VTQR_ESCAPEREDURateLimitInc_Nm  SystemSampleTime=-1  VariantActivationTime=update diagram  Latency=0  AutoFrameSizeCalculation=off
  VTQR_LHMREDURateLimitDec_Nm : tqr/TQR/Determine Torque Request/TorqueArbitrament/TorqueSmooth/Rear wheel rate limit determination1/VTQR_LHMREDURateLimitDec_Nm  SystemSampleTime=-1  VariantActivationTime=update diagram  Latency=0  AutoFrameSizeCalculation=off
  VTQR_LHMREDURateLimitInc_Nm : tqr/TQR/Determine Torque Request/TorqueArbitrament/TorqueSmooth/Rear wheel rate limit determination1/VTQR_LHMREDURateLimitInc_Nm  SystemSampleTime=-1  VariantActivationTime=update diagram  Latency=0  AutoFrameSizeCalculation=off
  VTQR_NORMALREDURateLimitDec_Nm : tqr/TQR/Determine Torque Request/TorqueArbitrament/TorqueSmooth/Rear wheel rate limit determination1/VTQR_NORMALREDURateLimitDec_Nm  SystemSampleTime=-1  VariantActivationTime=update diagram  Latency=0  AutoFrameSizeCalculation=off
  VTQR_NORMALREDURateLimitInc_Nm : tqr/TQR/Determine Torque Request/TorqueArbitrament/TorqueSmooth/Rear wheel rate limit determination1/VTQR_NORMALREDURateLimitInc_Nm  SystemSampleTime=-1  VariantActivationTime=update diagram  Latency=0  AutoFrameSizeCalculation=off
  VTQR_RrPreLoadTqIncDecSR_Nm : Subsystem  TreatAsAtomicUnit=on
  VTQR_SNOWREDURateLimitDec_Nm : tqr/TQR/Determine Torque Request/TorqueArbitrament/TorqueSmooth/Rear wheel rate limit determination1/VTQR_SNOWREDURateLimitDec_Nm  SystemSampleTime=-1  VariantActivationTime=update diagram  Latency=0  AutoFrameSizeCalculation=off
  VTQR_SNOWREDURateLimitInc_Nm : tqr/TQR/Determine Torque Request/TorqueArbitrament/TorqueSmooth/Rear wheel rate limit determination1/VTQR_SNOWREDURateLimitInc_Nm  SystemSampleTime=-1  VariantActivationTime=update diagram  Latency=0  AutoFrameSizeCalculation=off
  VTQR_SPORTREDURateLimitDec_Nm : tqr/TQR/Determine Torque Request/TorqueArbitrament/TorqueSmooth/Rear wheel rate limit determination1/VTQR_SPORTREDURateLimitDec_Nm  SystemSampleTime=-1  VariantActivationTime=update diagram  Latency=0  AutoFrameSizeCalculation=off
  VTQR_SPORTREDURateLimitInc_Nm : tqr/TQR/Determine Torque Request/TorqueArbitrament/TorqueSmooth/Rear wheel rate limit determination1/VTQR_SPORTREDURateLimitInc_Nm  SystemSampleTime=-1  VariantActivationTime=update diagram  Latency=0  AutoFrameSizeCalculation=off
  VTQR_TCSREDURateLimitDec_Nm : tqr/TQR/Determine Torque Request/TorqueArbitrament/TorqueSmooth/Rear wheel rate limit determination1/VTQR_TCSREDURateLimitDec_Nm  SystemSampleTime=-1  VariantActivationTime=update diagram  Latency=0  AutoFrameSizeCalculation=off
  VTQR_TCSREDURateLimitInc_Nm : tqr/TQR/Determine Torque Request/TorqueArbitrament/TorqueSmooth/Rear wheel rate limit determination1/VTQR_TCSREDURateLimitInc_Nm  SystemSampleTime=-1  VariantActivationTime=update diagram  Latency=0  AutoFrameSizeCalculation=off
  VTQR_VMCREDUTqIncDecSR_Nm : Subsystem  TreatAsAtomicUnit=on
  VTQR_RrRateLimitInc_Nm : Outport
  VTQR_RrRateLimitDec_Nm : Outport  Port=2
  wires:
  VTQD_TqTargetShaftSpd_rpm/1 -> [VTQD_TqTargetShaftSpd_rpm]
  Merge/1 -> Demux/1
  VTQD_TqSourceRr_enum/1 -> [VTQD_TqSourceRr_enum]
  VTQR_RrTqZeroTrans_enum/1 -> [VTQR_RrTqZeroTrans_enum]
  VTQD_LimpHomeAct_flg/1 -> [VTQD_LimpHomeAct_flg]
  VTQR_EVDriveMode_enum/1 -> [VTQR_EVDriveMode_enum]
  VDHP_ActAPSPosn_pct/1 -> [VDHP_ActAPSPosn_pct]
  VTQR_REDUWhlTqReqSmoothDelay_Nm/1 -> [VTQR_REDUWhlTqReqSmoothDelay_Nm]
  VTQD_EVDriveModeValid_flg/1 -> [VTQD_EVDriveModeValid_flg]
  VTQD_RegenMode_enum/1 -> [VTQD_RegenMode_enum]
  VVMC_ACCPedalOvrd_flg/1 -> [VVMC_ACCPedalOvrd_flg]
  VVMC_CCPedalOvrd_flg/1 -> [VVMC_CCPedalOvrd_flg]
  [VTQR_RrRDCActRateLimitInc_flg] -> Switch/2
  Demux/1 -> Switch/3
  VTQD_CreepPrLoadEnable_flg/1 -> [VTQD_CreepPrLoadEnable_flg]
  VTQD_PreLoadPreEn_flg/1 -> [VTQD_PreLoadPreEn_flg]
  VTQD_RDCActive_enum/1 -> [VTQD_RDCActive_enum]
  VTQR_NoABSREDUWhlTqReq_Nm/1 -> [VTQR_NoABSREDUWhlTqReq_Nm]
  VTQR_RampREDUWhlTqReq_Nm/1 -> [VTQR_RampREDUWhlTqReq_Nm]
  AND/1 -> [VTQR_RrRDCActRateLimitInc_flg]  "VTQR_RrRDCActRateLimitInc_flg"
  Constant12/1 -> Relational Operator2/2
  [VTQR_RampREDUWhlTqReq_Nm] -> Relational Operator2/1
  Equal2/1 -> AND/2
  Relational Operator2/1 -> AND/1
  Constant5/1 -> Equal2/2
  [VTQD_RDCActive_enum] -> Equal2/1
  VTQR_RrFirstOrderInpTq_Nm/1 -> [VTQR_RrFirstOrderInpTq_Nm]
  MTQR_AltRDCActiveREDUInc_Z_Nm/1 -> [VTQR_RDCActiveREDUInc_Nm]  "VTQR_RDCActiveREDUInc_Nm"
  Data Type Conversion/1 -> MTQR_AltRDCActiveREDUInc_Z_Nm/1
  [VTQD_RegenMode_enum] -> Data Type Conversion/1
  [VTQR_RDCActiveREDUInc_Nm] -> Switch/1
  [VVMC_ActMaxSlideRate_pct] -> MTQR_AltRDCActiveREDUInc_Z_Nm/2
  VTQD_PedAccTqEn_flg/1 -> [VTQD_PedAccTqEn_flg]
  VTQD_RegenTqLimitEn_flg/1 -> [VTQD_RegenTqLimitEn_flg]
  VVMC_ActMaxSlideRate_pct/1 -> [VVMC_ActMaxSlideRate_pct]
  [VTQR_VMCREDUTqDecSR_Nm] -> Switch7/1
  AND2/1 -> Switch7/2
  Constant6/1 -> AND2/2
  Demux/2 -> Switch7/3
  [VTQD_RegenTqLimitEn_flg] -> AND2/1
  VVMC_MSAWhlTqActive_flg/1 -> [VVMC_MSAWhlTqActive_flg]
  VINP_RrPTCSActive_flg/1 -> [VINP_RrPTCSActive_flg]
  VTQD_GearActualPosn_enum/1 -> [VTQD_GearActualPosn_enum]
  Equal/1 -> AND5/1
  Gain2/1 -> Switch8/3
  Constant20/1 -> Equal1/2
  [VTQD_GearActualPosn_enum] -> Equal1/1
  Constant18/1 -> Equal/2
  Constant19/1 -> AND5/2
  Gain3/1 -> Switch8/1
  [VTQD_GearActualPosn_enum] -> Equal/1
  Constant21/1 -> AND6/2
  Gain5/1 -> Switch9/1
  AND6/1 -> Switch9/2
  AND5/1 -> Switch8/2
  Gain4/1 -> Switch9/3
  Equal1/1 -> AND6/1
  Switch8/1 -> VTQR_RrRateLimitInc_Nm/1  "VTQR_RrRateLimitInc_Nm"
  Switch9/1 -> VTQR_RrRateLimitDec_Nm/1  "VTQR_RrRateLimitDec_Nm"
  Switch/1 -> [VTQR_OrigRrRateLimitInc_Nm]  "VTQR_OrigRrRateLimitInc_Nm"
  Switch7/1 -> [VTQR_OrigRrRateLimitDec_Nm]  "VTQR_OrigRrRateLimitDec_Nm"
  [VTQR_OrigRrRateLimitInc_Nm] -> Gain2/1
  [VTQR_OrigRrRateLimitInc_Nm] -> Gain5/1
  [VTQR_OrigRrRateLimitDec_Nm] -> Gain4/1
  [VTQR_OrigRrRateLimitDec_Nm] -> Gain3/1
  VTQD_IVIRockModeEn_flg/1 -> [VTQD_IVIRockModeEn_flg]
  VINP_IVISnowModeCmd_flg/1 -> [VINP_IVISnowModeCmd_flg]
  VTQD_RrShaftSpd_rpm/1 -> [VTQD_RrShaftSpd_rpm]
  VVMC_EstSlope_Deg/1 -> [VVMC_EstSlope_Deg]
  VTQD_VehActSpd_kph/1 -> [VTQD_VehActSpd_kph]
  VINP_ACCVehHoldReq_flg/1 -> [VINP_ACCVehHoldReq_flg]
  VPMM_DriveTrainSelect_enum/1 -> [VPMM_DriveTrainSelect_enum]
  VINP_VehicleType_enum/1 -> [VINP_VehicleType_enum]
  VVMC_ADASActive_flg/1 -> [VVMC_ADASActive_flg]
  VTQD_CoordWhlTqDemRr_Nm/1 -> [VTQD_CoordWhlTqDemRr_Nm]
  VINP_RearAxlTrqReqDrv_Nm/1 -> [VINP_RearAxlTrqReqDrv_Nm]
  VTQD_RrZeroPointIncDec_Nm/1 -> [VTQD_RrZeroPointIncDec_Nm]
  Logical Operator3/1 -> If3/1
  Relational Operator1/1 -> Logical Operator3/1
  [VTQR_RrTqZeroTrans_enum] -> Relational Operator1/1
  Constant4/1 -> Relational Operator1/2
  If3/1 -> VTQD_OutRrZeroPointIncDec_Nm/Action
  [VTQD_RrZeroPointIncDec_Nm] -> VTQD_OutRrZeroPointIncDec_Nm/1(VTQD_RrZeroPointIncDec_Nm)
  NOT2/1 -> AND8/2
  Constant9/1 -> Relational Operator8/2
  NOT3/1 -> AND8/3
  Relational Operator9/1 -> Logical Operator4/2
  [VVMC_CCPedalOvrd_flg] -> NOT3/1
  [VTQD_TqSourceRr_enum] -> Relational Operator8/1
  Constant30/1 -> Relational Operator9/2
  [VVMC_ACCPedalOvrd_flg] -> NOT2/1
  [VVMC_MSAWhlTqActive_flg] -> AND9/2
  [VTQD_TqSourceRr_enum] -> Relational Operator10/1
  [VTQD_CreepPrLoadEnable_flg] -> Logical Operator4/4
  [VTQD_TqSourceRr_enum] -> Relational Operator9/1
  AND9/1 -> Logical Operator4/3
  Logical Operator4/1 -> AND8/1
  [VTQD_PreLoadPreEn_flg] -> Logical Operator4/5
  Relational Operator10/1 -> AND9/1
  Constant7/1 -> Relational Operator10/2
  Relational Operator8/1 -> Logical Operator4/1
  [VTQD_PedAccTqEn_flg] -> Logical Operator4/6
  AND8/1 -> [VTQR_ADASCase_flg]
  [VTQD_CreepPrLoadEnable_flg] -> OR1/1
  [VTQD_PreLoadPreEn_flg] -> OR1/2
  OR1/1 -> [VTQR_PreLoadCase_flg]
  Logical Operator/1 -> If3/2
  [VTQR_ADASCase_flg] -> Logical Operator/1
  [VTQR_PreLoadCase_flg] -> Logical Operator/2
  [VTQD_CreepPrLoadEnable_flg] -> Logical Operator/3
  If3/2 -> VTQR_CreepREDUTqIncDecSR_Nm/Action
  [VTQR_REDUWhlTqReqSmoothDelay_Nm] -> VTQR_CreepREDUTqIncDecSR_Nm/1(VTQR_REDUWhlTqReqSmoothDelay_Nm)
  [VTQD_TqTargetShaftSpd_rpm] -> VTQR_CreepREDUTqIncDecSR_Nm/2(VTQD_TqTargetShaftSpd_rpm)
  VTQD_OutRrZeroPointIncDec_Nm/1(VTQD_OutRrZeroPointIncDec_Nm) -> [VTQD_OutRrZeroPointIncDec_Nm]  "VTQR_LHMREDURateLimitInc_Nm"
  VTQR_CreepREDUTqIncDecSR_Nm/1(VTQR_CreepREDUTqIncDecSR_Nm) -> [VTQR_CreepREDUTqIncDecSR_Nm]  "VTQR_CreepREDUTqIncDecSR_Nm"
  [VTQR_PreLoadCase_flg] -> Logical Operator5/2
  [VTQR_ADASCase_flg] -> Logical Operator5/1
  Logical Operator5/1 -> If3/3
  Logical Operator6/1 -> Logical Operator5/3
  [VTQD_CreepPrLoadEnable_flg] -> Logical Operator6/1
  If3/3 -> VTQR_RrPreLoadTqIncDecSR_Nm/Action
  [VTQR_REDUWhlTqReqSmoothDelay_Nm] -> VTQR_RrPreLoadTqIncDecSR_Nm/1(VTQR_REDUWhlTqReqSmoothDelay_Nm)
  [VTQD_TqTargetShaftSpd_rpm] -> VTQR_RrPreLoadTqIncDecSR_Nm/2(VTQD_TqTargetShaftSpd_rpm)
  VTQR_RrPreLoadTqIncDecSR_Nm/1(VTQR_RrPreLoadTqIncDecSR_Nm) -> [VTQR_RrPreLoadTqIncDecSR_Nm]  "VTQR_RrPreLoadTqIncDecSR_Nm"
  [VTQR_PreLoadCase_flg] -> Logical Operator9/1
  [VTQR_ADASCase_flg] -> Logical Operator8/1
  Logical Operator9/1 -> Logical Operator8/2
  Logical Operator8/1 -> If3/4
  [VTQR_REDUWhlTqReqSmoothDelay_Nm] -> VTQR_VMCREDUTqIncDecSR_Nm/1(VTQR_REDUWhlTqReqSmoothDelay_Nm)
  [VTQD_TqTargetShaftSpd_rpm] -> VTQR_VMCREDUTqIncDecSR_Nm/2(VTQD_TqTargetShaftSpd_rpm)
  VTQR_VMCREDUTqIncDecSR_Nm/1(VTQR_VMCREDUTqIncDecSR_Nm) -> [VTQR_VMCREDUTqIncDecSR_Nm]  "VTQR_VMCREDUTqIncDecSR_Nm"
  VTQR_VMCREDUTqIncDecSR_Nm/2(VTQR_VMCREDUTqDecSR_Nm) -> [VTQR_VMCREDUTqDecSR_Nm]
  [VTQD_OutRrZeroPointIncDec_Nm] -> Merge/1
  [VTQR_CreepREDUTqIncDecSR_Nm] -> Merge/2
  [VTQR_RrPreLoadTqIncDecSR_Nm] -> Merge/3
  [VTQR_VMCREDUTqIncDecSR_Nm] -> Merge/4
  [VTQD_RegenMode_enum] -> VTQR_SPORTREDURateLimitDec_Nm/3
  [VTQR_EVDriveMode_enum] -> Equal23/1
  Logical Operator12/1 -> If5/1
  [VTQR_REDUWhlTqReqSmoothDelay_Nm] -> VTQR_LHMREDURateLimitDec_Nm/1
  Constant26/1 -> Equal24/2
  [VTQD_RegenMode_enum] -> VTQR_NORMALREDURateLimitDec_Nm/3
  [VTQD_LimpHomeAct_flg] -> Logical Operator12/1
  [VTQR_EVDriveMode_enum] -> Equal25/1
  Logical Operator10/1 -> If4/1
  Constant27/1 -> Equal25/2
  Constant22/1 -> Equal20/2
  [VTQR_REDUWhlTqReqSmoothDelay_Nm] -> VTQR_SNOWREDURateLimitInc_Nm/3
  [VTQR_REDUWhlTqReqSmoothDelay_Nm] -> VTQR_SPORTREDURateLimitDec_Nm/1
  Logical Operator1/1 -> If4/2
  [VINP_RearAxlTrqReqDrv_Nm] -> " Relational Operator8"/2
  [VTQD_RegenMode_enum] -> VTQR_ECOREDURateLimitDec_Nm/3
  [VINP_RrPTCSActive_flg] -> Logical Operator2/1
  [VTQD_TqTargetShaftSpd_rpm] -> VTQR_SPORTREDURateLimitDec_Nm/2
  [VINP_VehicleType_enum] -> Equal8/1
  Equal8/1 -> Logical Operator2/2
  Logical Operator2/1 -> If5/2
  VTQR_ESCAPEREDURateLimitDec_Nm/1 -> [VTQR_ESCAPEREDURateLimitDec_Nm]  "VTQR_ESCAPEREDURateLimitDec_Nm"
  If5/3 -> VTQR_ESCAPEREDURateLimitDec_Nm/Action
  [VTQR_REDUWhlTqReqSmoothDelay_Nm] -> VTQR_ECOREDURateLimitDec_Nm/1
  If4/5 -> VTQR_NORMALREDURateLimitInc_Nm/Action
  [VTQD_CoordWhlTqDemRr_Nm] -> " Relational Operator1"/1
  [VTQR_REDUWhlTqReqSmoothDelay_Nm] -> VTQR_SPORTREDURateLimitInc_Nm/4
  Constant29/1 -> Equal8/2
  " Relational Operator1"/1 -> Logical Operator2/3
  [VTQD_TqTargetShaftSpd_rpm] -> VTQR_SNOWREDURateLimitInc_Nm/2
  If4/3 -> VTQR_ESCAPEREDURateLimitInc_Nm/Action
  [VTQD_TqTargetShaftSpd_rpm] -> VTQR_LHMREDURateLimitInc_Nm/2
  [VINP_RrPTCSActive_flg] -> Logical Operator1/1
  [VTQD_CoordWhlTqDemRr_Nm] -> " Relational Operator8"/1
  " Relational Operator8"/1 -> Logical Operator1/3
  Equal7/1 -> Logical Operator1/2
  Constant25/1 -> Equal7/2
  [VINP_VehicleType_enum] -> Equal7/1
  VTQR_NORMALREDURateLimitDec_Nm/1 -> [VTQR_NORMALREDURateLimitDec_Nm]  "VTQR_NORMALREDURateLimitDec_Nm"
  Logical Operator13/1 -> Logical Operator12/2
  [VDHP_ActAPSPosn_pct] -> VTQR_SNOWREDURateLimitInc_Nm/1
  Equal25/1 -> If5/5
  [VINP_IVISnowModeCmd_flg] -> If4/4
  If5/6 -> VTQR_ECOREDURateLimitDec_Nm/Action
  [VTQD_IVIRockModeEn_flg] -> If4/3
  If5/1 -> VTQR_LHMREDURateLimitDec_Nm/Action
  Constant24/1 -> Equal23/2
  [VTQD_IVIRockModeEn_flg] -> If5/3
  [VTQR_EVDriveMode_enum] -> Equal27/1
  If5/2 -> VTQR_TCSREDURateLimitDec_Nm/Action
  [VTQR_REDUWhlTqReqSmoothDelay_Nm] -> VTQR_NORMALREDURateLimitDec_Nm/1
  VTQR_NORMALREDURateLimitInc_Nm/1 -> [VTQR_NORMALREDURateLimitInc_Nm]  "VTQR_NORMALREDURateLimitInc_Nm"
  VTQR_SPORTREDURateLimitInc_Nm/1 -> [VTQR_SPORTREDURateLimitInc_Nm]  "VTQR_SPORTREDURateLimitInc_Nm"
  VTQR_LHMREDURateLimitInc_Nm/1 -> [VTQR_LHMREDURateLimitInc_Nm]  "VTQR_LHMREDURateLimitInc_Nm"
  If4/6 -> VTQR_ECOREDURateLimitInc_Nm/Action
  VTQR_TCSREDURateLimitInc_Nm/1 -> [VTQR_TCSREDURateLimitInc_Nm]  "VTQR_TCSREDURateLimitInc_Nm"
  VTQR_SNOWREDURateLimitInc_Nm/1 -> [VTQR_SNOWREDURateLimitInc_Nm]  "VTQR_SNOWREDURateLimitInc_Nm"
  VTQR_ESCAPEREDURateLimitInc_Nm/1 -> [VTQR_ESCAPEREDURateLimitInc_Nm]  "VTQR_ESCAPEREDURateLimitInc_Nm"
  [VTQD_RegenMode_enum] -> VTQR_ECOREDURateLimitInc_Nm/3
  [VTQD_RrShaftSpd_rpm] -> VTQR_ESCAPEREDURateLimitDec_Nm/2
  [VTQD_RrShaftSpd_rpm] -> VTQR_ESCAPEREDURateLimitInc_Nm/2
  [VDHP_ActAPSPosn_pct] -> VTQR_ESCAPEREDURateLimitInc_Nm/1
  Equal20/1 -> If4/6
  If4/2 -> VTQR_TCSREDURateLimitInc_Nm/Action
  [VTQD_TqTargetShaftSpd_rpm] -> VTQR_NORMALREDURateLimitDec_Nm/2
  If5/5 -> VTQR_NORMALREDURateLimitDec_Nm/Action
  VTQR_SPORTREDURateLimitDec_Nm/1 -> [VTQR_SPORTREDURateLimitDec_Nm]  "VTQR_SPORTREDURateLimitDec_Nm"
  [VTQD_LimpHomeAct_flg] -> Logical Operator10/1
  [VTQD_TqTargetShaftSpd_rpm] -> VTQR_SNOWREDURateLimitDec_Nm/2
  [VTQR_REDUWhlTqReqSmoothDelay_Nm] -> VTQR_ESCAPEREDURateLimitDec_Nm/1
  VTQR_SNOWREDURateLimitDec_Nm/1 -> [VTQR_SNOWREDURateLimitDec_Nm]  "VTQR_SNOWREDURateLimitDec_Nm"
  [VTQD_TqTargetShaftSpd_rpm] -> VTQR_TCSREDURateLimitDec_Nm/2
  If5/4 -> VTQR_SNOWREDURateLimitDec_Nm/Action
  Equal24/1 -> If5/6
  If5/7 -> VTQR_SPORTREDURateLimitDec_Nm/Action
  [VTQD_EVDriveModeValid_flg] -> Logical Operator11/1
  [VINP_RearAxlTrqReqDrv_Nm] -> " Relational Operator1"/2
  VTQR_TCSREDURateLimitDec_Nm/1 -> [VTQR_TCSREDURateLimitDec_Nm]  "VTQR_TCSREDURateLimitDec_Nm"
  If4/7 -> VTQR_SPORTREDURateLimitInc_Nm/Action
  [VTQR_EVDriveMode_enum] -> Equal21/1
  [VINP_IVISnowModeCmd_flg] -> If5/4
  VTQR_ECOREDURateLimitInc_Nm/1 -> [VTQR_ECOREDURateLimitInc_Nm]  "VTQR_ECOREDURateLimitInc_Nm"
  [VTQD_RegenMode_enum] -> VTQR_NORMALREDURateLimitInc_Nm/3
  VTQR_ECOREDURateLimitDec_Nm/1 -> [VTQR_ECOREDURateLimitDec_Nm]  "VTQR_ECOREDURateLimitDec_Nm"
  [VTQD_TqTargetShaftSpd_rpm] -> VTQR_ECOREDURateLimitDec_Nm/2
  [VTQD_TqTargetShaftSpd_rpm] -> VTQR_SPORTREDURateLimitInc_Nm/2
  [VTQR_REDUWhlTqReqSmoothDelay_Nm] -> VTQR_TCSREDURateLimitDec_Nm/1
  [VDHP_ActAPSPosn_pct] -> VTQR_LHMREDURateLimitInc_Nm/1
  If4/4 -> VTQR_SNOWREDURateLimitInc_Nm/Action
  [VDHP_ActAPSPosn_pct] -> VTQR_TCSREDURateLimitInc_Nm/1
  [VTQD_TqTargetShaftSpd_rpm] -> VTQR_ECOREDURateLimitInc_Nm/2
  [VTQD_TqTargetShaftSpd_rpm] -> VTQR_TCSREDURateLimitInc_Nm/2
  [VDHP_ActAPSPosn_pct] -> VTQR_ECOREDURateLimitInc_Nm/1
  Equal21/1 -> If4/5
  If4/1 -> VTQR_LHMREDURateLimitInc_Nm/Action
  [VTQR_REDUWhlTqReqSmoothDelay_Nm] -> VTQR_ECOREDURateLimitInc_Nm/4
  [VDHP_ActAPSPosn_pct] -> VTQR_NORMALREDURateLimitInc_Nm/1
  VTQR_LHMREDURateLimitDec_Nm/1 -> [VTQR_LHMREDURateLimitDec_Nm]  "VTQR_LHMREDURateLimitDec_Nm"
  Logical Operator11/1 -> Logical Operator10/2
  Equal23/1 -> If4/7
  [VDHP_ActAPSPosn_pct] -> VTQR_SPORTREDURateLimitInc_Nm/1
  Constant23/1 -> Equal21/2
  [VTQR_REDUWhlTqReqSmoothDelay_Nm] -> VTQR_NORMALREDURateLimitInc_Nm/4
  [VTQD_EVDriveModeValid_flg] -> Logical Operator13/1
  [VTQR_EVDriveMode_enum] -> Equal24/1
  [VTQD_TqTargetShaftSpd_rpm] -> VTQR_LHMREDURateLimitDec_Nm/2
  Equal27/1 -> If5/7
  [VTQD_RegenMode_enum] -> VTQR_SPORTREDURateLimitInc_Nm/3
  [VTQD_TqTargetShaftSpd_rpm] -> VTQR_NORMALREDURateLimitInc_Nm/2
  [VTQR_REDUWhlTqReqSmoothDelay_Nm] -> VTQR_SNOWREDURateLimitDec_Nm/1
  Constant28/1 -> Equal27/2
  [VTQR_EVDriveMode_enum] -> Equal20/1
  [VTQR_LHMREDURateLimitInc_Nm] -> Merge4/1
  [VTQR_NORMALREDURateLimitInc_Nm] -> Merge4/5
  [VTQR_ECOREDURateLimitInc_Nm] -> Merge4/6
  [VTQR_SNOWREDURateLimitInc_Nm] -> Merge4/4
  [VTQR_TCSREDURateLimitInc_Nm] -> Merge4/2
  [VTQR_ESCAPEREDURateLimitInc_Nm] -> Merge4/3
  [VTQR_EVDriveMode_enum] -> Detect Change/1
  Merge4/1 -> Switch4/3
  Delay/1 -> Switch4/1
  SR_Latch1/1 -> Switch4/2, [VTQR_RrDrModIncLatch_flg]
  [VTQR_RrDrModChangeReset_flg] -> SR_Latch1/2
  Detect Change/1 -> SR_Latch1/1
  [VTQR_SPORTREDURateLimitInc_Nm] -> Merge4/7
  Switch4/1 -> Delay/1, [VTQR_OriREDURateLimitInc_Nm]  "VTQR_OriREDURateLimitInc_Nm"
  [VTQR_LHMREDURateLimitDec_Nm] -> Merge5/1
  Switch5/1 -> Delay2/1, [VTQR_REDURateLimitDec_Nm]  "VTQR_REDURateLimitDec_Nm"
  [VTQR_TCSREDURateLimitDec_Nm] -> Merge5/2
  [VTQR_NORMALREDURateLimitDec_Nm] -> Merge5/5
  [VTQR_SNOWREDURateLimitDec_Nm] -> Merge5/4
  [VTQR_SPORTREDURateLimitDec_Nm] -> Merge5/7
  [VTQR_ESCAPEREDURateLimitDec_Nm] -> Merge5/3
  SR_Latch2/1 -> Switch5/2, [VTQR_RrDrModDecLatch_flg]
  [VTQR_EVDriveMode_enum] -> Detect Change1/1
  Merge5/1 -> Switch5/3
  [VTQR_ECOREDURateLimitDec_Nm] -> Merge5/6
  Delay2/1 -> Switch5/1
  [VTQR_RrDrModChangeReset_flg] -> SR_Latch2/2
  Detect Change1/1 -> SR_Latch2/1
  [VPMM_DriveTrainSelect_enum] -> Equal5/1
  Equal4/1 -> AND7/3
  Equal6/1 -> SR_Latch3/2
  Constant14/1 -> Equal5/2
  [VVMC_EstSlope_Deg] -> Equal3/1
  [VTQR_OriREDURateLimitInc_Nm] -> Max1/1
  AND7/1 -> SR_Latch3/1  "VTQR_ACCHoldPdovrdInc_flg"
  Detect Increase/1 -> AND7/6
  Constant13/1 -> AND7/5
  SR_Latch3/1 -> Switch10/2
  Max1/1 -> Switch10/3
  [VVMC_ACCPedalOvrd_flg] -> AND7/1
  Constant/1 -> Equal3/2
  Equal5/1 -> AND7/7
  Equal3/1 -> AND7/2
  Switch10/1 -> [VTQR_REDURateLimitInc_Nm]  "VTQR_REDURateLimitInc_Nm"
  [VVMC_ADASActive_flg] -> AND7/4
  [VTQD_VehActSpd_kph] -> Equal4/1
  [VTQR_OriREDURateLimitInc_Nm] -> Max/1
  [VTQR_OriREDURateLimitInc_Nm] -> Equal6/1
  Constant16/1 -> Max/2
  Constant15/1 -> Equal6/2
  [VINP_ACCVehHoldReq_flg] -> Detect Increase/1
  Constant17/1 -> Max1/2
  Max/1 -> Switch10/1
  Constant11/1 -> Equal4/2
  Relational Operator6/1 -> AND4/1
  Abs4/1 -> Relational Operator6/1
  AND4/1 -> OR2/2
  [VTQR_RrFirstOrderInpTq_Nm] -> Add/2
  Delay1/1 -> Add1/1
  Constant8/1 -> Relational Operator6/2
  [VTQR_RrFirstOrderInpTq_Nm] -> Delay1/1
  Relational Operator5/1 -> OR2/1
  Add1/1 -> Abs4/1
  Delay4/1 -> OR3/2
  OR3/1 -> AND4/2
  [VTQR_NoABSREDUWhlTqReq_Nm] -> Add/1
  Add/1 -> Abs/1
  OR2/1 -> [VTQR_RrDrModChangeReset_flg]  "VTQR_RrDrModChangeReset_flg"
  Delay3/1 -> OR3/1
  Abs/1 -> Relational Operator5/1
  [VTQR_RrDrModIncLatch_flg] -> Delay3/1
  Constant2/1 -> Relational Operator5/2
  [VTQR_RrDrModDecLatch_flg] -> Delay4/1
  [VTQR_RrFirstOrderInpTq_Nm] -> Add1/2
  [VTQR_REDURateLimitDec_Nm] -> Mux/2
  [VTQR_REDURateLimitInc_Nm] -> Mux/1
  Mux/1 -> [VTQR_DriveModeTqIncDec_Nm]
  If3/4 -> VTQR_VMCREDUTqIncDecSR_Nm/Action
  If3/5 -> Drive mode/Action
  [VTQR_DriveModeTqIncDec_Nm] -> Drive mode/1(VTQR_DriveModeTqIncDec_Nm)
  Drive mode/1(VTQR_OutDriveModeTqIncDec_Nm) -> [VTQR_OutDriveModeTqIncDec_Nm]  "VTQR_OutDriveModeTqIncDec_Nm"
  [VTQR_OutDriveModeTqIncDec_Nm] -> Merge/5
  [VVMC_EstSlope_Deg] -> VTQR_CreepREDUTqIncDecSR_Nm/3(VVMC_EstSlope_Deg)
